simulink model "SF5_9_4_jm0012_2"  (R2016b)
settings: Solver=VariableStepAuto  StartTime=0.0  StopTime=10.0  RelTol=1e-3
settings Model: Creator=amyyang  LastModifiedBy=amyyang

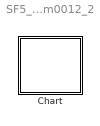
== system SF5_9_4_jm0012_2 ==
  Chart : Stateflow chart  TreatAsAtomicUnit=on

== stateflow chart SF5_9_4_jm0012_2/Chart ==
  state A [parallel]
    settings: executionOrder=1
    state A1
    state A2
    (default) -> A1
    A1 -> A2 : /Event1
    A2 -> A1
  state B [parallel]
    settings: executionOrder=2
    state B1
    state B2
    (default) -> B1
    B1 -> B2 : Event1
    B2 -> B1
  events: Event1 local FUNCTION_CALL_EVENT
